simulink model "varSS1_calc_add_sub"  (R2025a)
settings: Solver=VariableStepAuto  StartTime=0.0  StopTime=10.0  RelTol=1e-3
settings Model: Creator=z004f2se  LastModifiedBy=z004f2se

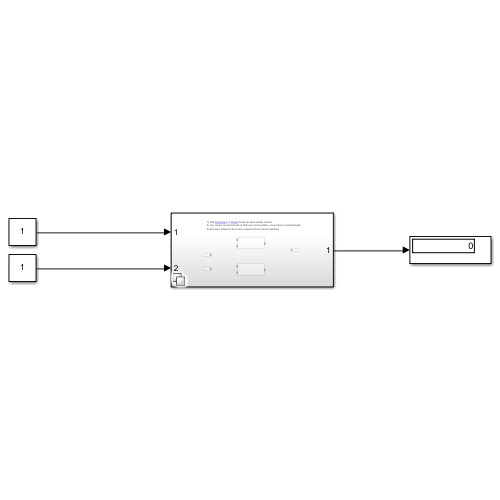
[thumbnail: Simulink's stored preview of the top-level diagram]
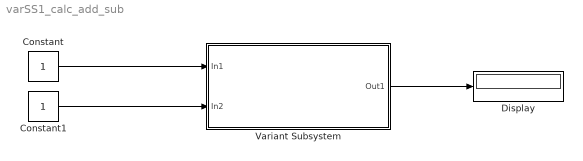
== system varSS1_calc_add_sub ==
  Constant : Constant
  Constant1 : Constant
  Display : Display
  Variant Subsystem : Subsystem  Variant=on
  wires:
  Constant/1 -> Variant Subsystem/1(In1)
  Constant1/1 -> Variant Subsystem/2(In2)
  Variant Subsystem/1(Out1) -> Display/1

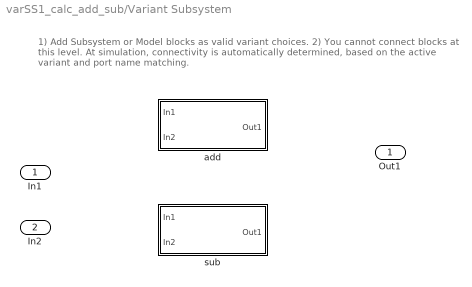
== system varSS1_calc_add_sub/Variant Subsystem ==
  note: 1) Add Subsystem or Model blocks as valid variant choices.
      | 2) You cannot connect blocks at this level. At simulation, connectivity is automatically
      | determined, based on the active variant and port name matching.
  In1 : Inport
  In2 : Inport  Port=2
  add : Subsystem  VariantControl=op==1
  sub : Subsystem  VariantControl=op==2
  Out1 : Outport

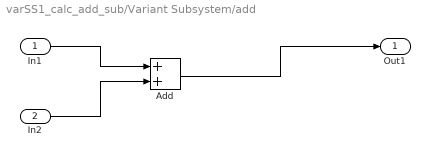
== system varSS1_calc_add_sub/Variant Subsystem/add ==
  In1 : Inport
  In2 : Inport  Port=2
  Add : Sum
  Out1 : Outport
  wires:
  In1/1 -> Add/1
  In2/1 -> Add/2
  Add/1 -> Out1/1

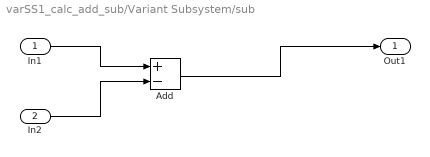
== system varSS1_calc_add_sub/Variant Subsystem/sub ==
  In1 : Inport
  In2 : Inport  Port=2
  Add : Sum  Inputs=+-
  Out1 : Outport
  wires:
  Add/1 -> Out1/1
  In1/1 -> Add/1
  In2/1 -> Add/2
